simulink model "platform"  (Simulink 8.8)
settings: Solver=ode4  StartTime=0.0  StopTime=500  FixedStep=0.05  RelTol=1e-3  EnableMultiTasking=on
settings Model: Creator=Furao  LastModifiedBy=Furao
settings DataIOCC: SignalLoggingName=sigsOut
settings OptimizationCC: LifeSpan=auto
settings DebuggingCC: SaveWithParameterizedLinksMsg=none  SignalResolutionControl=TryResolveAllWithWarning  MultiTaskDSMMsg=warning  MultiTaskCondExecSysMsg=none  FcnCallInpInsideContextMsg=error  StateNameClashWarn=none  SFUnexpectedBacktrackingDiag=error  SFNoUnconditionalDefaultTransitionDiag=error  SFExecutionAtInitializationDiag=warning
settings HardwareCC: TargetUnknown=on
settings GRTTargetCC: GeneratePreprocessorConditionals=Use local settings

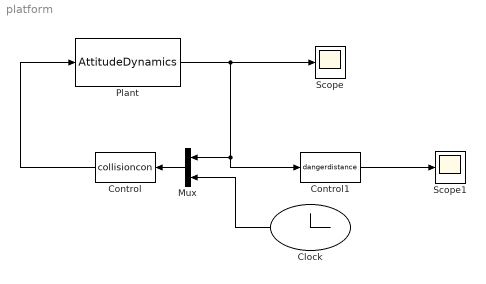
== system platform ==
  Clock : Clock
  Control : MATLABFcn  MATLABFcn=collisioncon
  Control1 : MATLABFcn  MATLABFcn=dangerdistance
  Mux : Mux  Inputs=2
  Plant : S-Function  FunctionName=AttitudeDynamics  SFunctionDeploymentMode=off  EnableBusSupport=off
  Scope : Scope
  Scope1 : Scope
  wires:
  Plant/1 -> Scope/1, Control1/1, Mux/1
  Control/1 -> Plant/1
  Control1/1 -> Scope1/1
  Mux/1 -> Control/1
  Clock/1 -> Mux/2
